simulink model "boat_dynamics_model"  (R2025a)
settings: Solver=ode4  StartTime=0.0  StopTime=15  FixedStep=Ts_sim  RelTol=1e-3
values from neighbouring files (symbols this model uses):
  ctrl_params =     [boat_controller_parameters.mat]    (also in setup_MDL.m = boat_controller_parameters())
  plant_params = boat_model_parameters_4dof()    [setup_MDL.m]
  trim =     [last_trim.mat]    (also in setup_RL.m = data.trim; tmp_trim_4dof.mat)
  u0 = u0(:)    [find_A_B_LQR.m]    (also in setup_MDL.m = trim.u0; setup_RL.m = trim.u0; tmp_continuous_controller.mat = [4.86274582601 4.86274582601 5.08309482386 4.40845063905]; tmp_discrete_augumented_LQI_controller.mat = [4.86274582601 4.86274582601 5.08309482386])
  x0 = x0(:)    [find_A_B_LQR.m]    (also in setup_MDL.m = trim.x0; setup_RL.m = trim.x0; tmp_continuous_controller.mat = [0 2.5 -0.1 0 0 0 0 0 0 0 4.86274582601 4.86274582601 ... (1; tmp_discrete_controller.mat = [0 2.5 -0.1 0 0 0 0 0 0 0 4.86274582601 4.86274582601 ... (1)
undefined symbols (not defined in the file or in its folder): Ts_sim
libraries: simulink_extras x4, sim3dlib x2, rllib x1
(part 1 of 2)
settings Model: Creator=brzan  LastModifiedBy=brzan

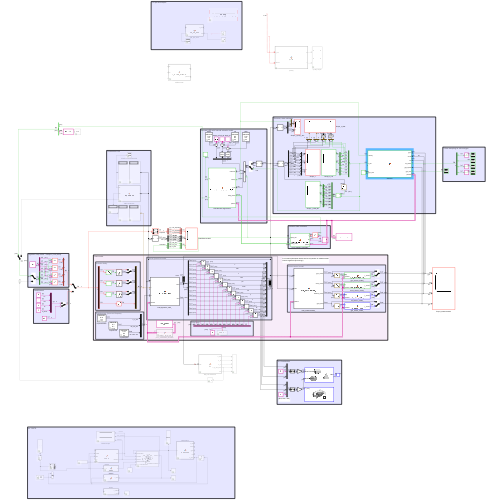
[thumbnail: Simulink's stored preview of the top-level diagram]
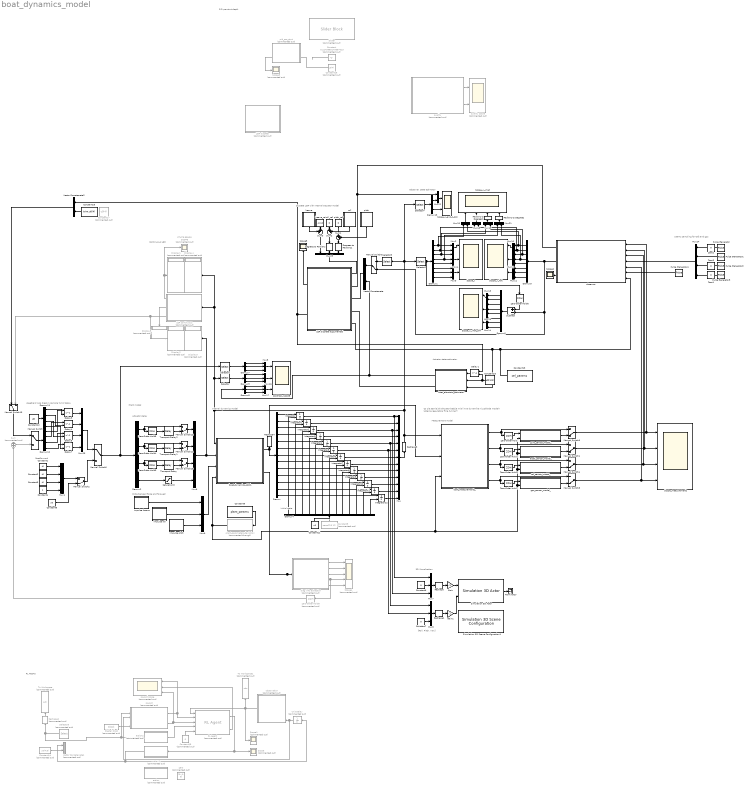
== system boat_dynamics_model ==
  note: 100ms sampling for tofs and gps
  note: Actuator state estimator
  note: PID per strut depth
  note: Plant model
  note: Actuator delay
  note: Algebraic loop break 1 sample (1ms) delay
  note: RL TESTS
  note: Observer, state estimator
  note: Co sie stanie jak aktuator bedzie mial inna dynamike niz zaklada model?
      | Uczenie regulatora (fine tuning?)
  note: Discrete LQR with Internal actuator model
  note: Continuous LQR
  note: Feedforward
  note: Measurement model
  note: Internal dynamics model
  note: Initial state
  note: Disturbances (force and forques)
  note: 3D Visualization
  note: [Roll, Pitch, Yaw]
  CONTROL SCOPE : Scope  NumInputPorts=3
      settings: ActiveDisplayYMinimum=-5.0548217064817056  ActiveDisplayYMaximum=7.8217886254018625  DataLoggingVariableName=ScopeAction
  Constant : Constant  Commented=on  Value=0.2275960170697013
  Constant1 : Constant  Value=-6
  Constant10 : Constant  Value=u0(1:3)  VectorParams1D=off
  Constant11 : Constant  Value=x0  VectorParams1D=off
  Constant12 : Constant  Value=u0  VectorParams1D=off
  Constant13 : Constant  Value=ctrl_params  VectorParams1D=off  OutDataTypeStr=Bus: ctrl_params_bus
  Constant14 : Constant  Commented=on  Value=u0(4:5)  VectorParams1D=off
  Constant15 : Constant  Commented=on  Value=0
  Constant16 : Constant  Commented=on  Value=u0(4)
  Constant17 : Constant  Commented=on  Value=u0(4)  VectorParams1D=off
  Constant18 : Constant  Value=trim.u0(4)  VectorParams1D=off
  Constant2 : Constant  Value=-6
  Constant3 : Constant  Value=-6
  Constant4 : Constant
  Constant5 : Constant  Commented=on  Value=zeros([13 1])  VectorParams1D=off
  Constant6 : Constant  Value=0
  Constant7 : Constant  Value=0
  Constant8 : Constant  Value=u0
  Constant9 : Constant  Value=plant_params  VectorParams1D=off  OutDataTypeStr=Bus: plant_params_bus
  Degrees to Radians : simulink_extras/Transformations/Degrees to Radians
  Degrees to Radians1 : simulink_extras/Transformations/Degrees to Radians
  Delay{1,3..5,7} (5 alike) : Delay  DelayLength=1  InitialConditionSource=Input port  SampleTime=Ts_sim
      settings: InputPortMap=u0,p4
  Demux : Demux  Outputs=13
  Demux1 : Demux  Outputs=8
  Demux11 : Demux
  Demux12 : Demux
  Demux13 : Demux  Outputs=2
  Demux2 : Demux
  Demux3 : Demux  Outputs=3
  Demux4 : Demux  Outputs=13
  Demux5 : Demux  Outputs=8
  Demux6 : Demux  Outputs=8
  Demux7 : Demux  Outputs=3
  Demux8 : Demux  Outputs=3
  Digital Clock : DigitalClock  Commented=on  SampleTime=0.01
  Display{1..5} (5 alike) : Display  Commented=on
  Gain : Gain  Gain=-1
  Gain1 : Gain  Gain=-1
  Impulse heave : Subsystem  mask{start=10, duration=2, amplitude=0}
      mask prompts: start "Start time"; duration "Duration time"; amplitude "Impulse amplitude"
      mask Display:
      | disp([ ...
      |     "IMPULSE"; ...
      |     'S ', ...
      |     num2str(get_param(gcb, 'start')); ...
      |     'D ', ...
      |     num2str(get_param(gcb, "duration")); ...
      |     'A ', ...
      |     num2str(get_param(gcb, "amplitude")) ...
      | ]);
  Impulse pitch : Subsystem  mask{start=10, duration=2, amplitude=0}
      mask prompts: start "Start time"; duration "Duration time"; amplitude "Impulse amplitude"
      mask Display:
      | disp([ ...
      |     "IMPULSE"; ...
      |     'S ', ...
      |     num2str(get_param(gcb, 'start')); ...
      |     'D ', ...
      |     num2str(get_param(gcb, "duration")); ...
      |     'A ', ...
      |     num2str(get_param(gcb, "amplitude")) ...
      | ]);
  Impulse roll : Subsystem  mask{start=3, duration=7, amplitude=0.5}
      mask prompts: start "Start time"; duration "Duration time"; amplitude "Impulse amplitude"
      mask Display:
      | disp([ ...
      |     "IMPULSE"; ...
      |     'S ', ...
      |     num2str(get_param(gcb, 'start')); ...
      |     'D ', ...
      |     num2str(get_param(gcb, "duration")); ...
      |     'A ', ...
      |     num2str(get_param(gcb, "amplitude")) ...
      | ]);
  Integrator : Integrator  InitialConditionSource=external  InitialCondition=-0.11
  Integrator{1,3..12} (11 alike) : Integrator  InitialConditionSource=external
  Integrator2 : Integrator  InitialConditionSource=external  InitialCondition=deg2rad(3)
  LQR continuous : MATLAB Function  Commented=on  TreatAsAtomicUnit=on
  LQR discrete : MATLAB Function  Commented=on  TreatAsAtomicUnit=on  SystemSampleTime=ctrl_params.Ts
  LQR discrete augumented : MATLAB Function  TreatAsAtomicUnit=on  SystemSampleTime=ctrl_params.Ts
  Manual Switch : ManualSwitch
  Manual Switch{1..5,8,10..12} (9 alike) : ManualSwitch  CurrentSetting=0
  Manual Switch13 : ManualSwitch
  Manual Switch6 : ManualSwitch
  Mux : Mux  Inputs=13
  Mux{1,6,23..24} (4 alike) : Mux
  Mux{2,10,13,18..22} (8 alike) : Mux  Inputs=2
  Mux{3..5,7..9,11..12,14..17,25} (13 alike) : Mux  Inputs=3
  Pulse Generator{,1..4} (5 alike) : DiscretePulseGenerator  Period=10  SampleTime=ctrl_params.Ts
  RL Agent : rllib/RL Agent  Commented=on  Agent=agentObj  ExternalActionAsInput=on  ProvideLastAction=off  ProvideCumRwd=on  TreatAsDirectFeedthrough=on  UseStrictObservationDataTypes=off
  Radians to Degrees : simulink_extras/Transformations/Radians to Degrees
  Radians to Degrees1 : simulink_extras/Transformations/Radians to Degrees
  Reshape : Reshape  OutputDimensionality=Row vector (2-D)
  Reshape1 : Reshape  OutputDimensionality=Row vector (2-D)
  Reshape2 : Reshape  Commented=on
  Reshape3 : Reshape  OutputDimensionality=Column vector (2-D)
  Reshape4 : Reshape  OutputDimensionality=Column vector (2-D)
  STATE ERROR SCOPE : Scope  Commented=on
      settings: ActiveDisplayYMinimum=-0.17004569092279864  ActiveDisplayYMaximum=0.25579071640803624  DataLoggingVariableName=ScopeData3
  Saturation3 : Saturate  UpperLimit=20  LowerLimit=0
  Scope : Scope  Commented=on
      settings: ActiveDisplayYMinimum=-2.4199088465030929  ActiveDisplayYMaximum=1.3794615097714347  DataLoggingVariableName=ScopeData2
  Scope1 : Scope  Commented=on
      settings: ActiveDisplayYMinimum=0.99404961030066707  ActiveDisplayYMaximum=1.0007752200523612  DataLoggingVariableName=ScopeData4
  Scope2 : Scope
      settings: ActiveDisplayYMinimum=-7.4600755666939691E-5  ActiveDisplayYMaximum=0.00062285522635525655  DataLoggingVariableName=ScopeData11
  Scope3 : Scope  Commented=on
      settings: ActiveDisplayYMinimum=-0.14108639149516483  ActiveDisplayYMaximum=0.0051605981146346652  DataLoggingVariableName=ScopeData12
  Scope4 : Scope  Commented=on  NumInputPorts=5
      settings: ActiveDisplayYMinimum=-0.58327189745525043  ActiveDisplayYMaximum=0.17485807514493268  DataLoggingVariableName=ScopeData13
  Scope5 : Scope
      settings: ActiveDisplayYMinimum=-0.22138752196784806  ActiveDisplayYMaximum=0.42850292012780228  DataLoggingVariableName=ScopeData6
  Scope_measurements : Scope  NumInputPorts=4
      settings: ActiveDisplayString=4  ActiveDisplayYMinimum=0.421125  ActiveDisplayYMaximum=2.9298750000000005
  Scope_x : Scope  NumInputPorts=3
      settings: ActiveDisplayYMinimum=-0.13106117710441487  ActiveDisplayYMaximum=0.06992887382000551
  Scope_x_and_z_dot : Scope  NumInputPorts=2
      settings: ActiveDisplayYMinimum=0.30889257492581745  ActiveDisplayYMaximum=2.8807711117217907  DataLoggingVariableName=ScopeData10
  Scope_x_hat : Scope  NumInputPorts=3
      settings: ActiveDisplayYMinimum=-0.12339067146341488  ActiveDisplayYMaximum=0.04600825658737881  DataLoggingVariableName=ScopeObservation
  Scope_x_xhat : Scope  NumInputPorts=4
      settings: ActiveDisplayYMinimum=-0.10922860786142216  ActiveDisplayYMaximum=-0.0926378252846192  DataLoggingVariableName=ScopeData7
  Scope_x_xhat_diff : Scope  NumInputPorts=3
      settings: ActiveDisplayYMinimum=-0.017709281074984293  ActiveDisplayYMaximum=0.023978409304645298  DataLoggingVariableName=ScopeData5
  Selector : Selector  InputPortWidth=13  IndexOptions=Index vector (dialog)  Indices=[11 12 13]  OutputSizes=1
  Selector1 : Selector  InputPortWidth=4  IndexOptions=Index vector (dialog)  Indices=[1 2 3]  OutputSizes=1
  Selector2 : Selector  InputPortWidth=13  IndexOptions=Index vector (dialog)  Indices=[3 4 5 6 7 8 9 10]  OutputSizes=1
  Selector3 : Selector  InputPortWidth=13  IndexOptions=Index vector (dialog)  Indices=[3 4 5 6 7 8 9 10]  OutputSizes=1
  Selector5 : Selector  Commented=on  InputPortWidth=5  IndexOptions=Index vector (dialog)  Indices=[1 2 3]  OutputSizes=1
  Selector7 : Selector  InputPortWidth=13  IndexOptions=Index vector (dialog)  Indices="[ 2  4 ]"  OutputSizes=1
  Simulation 3D Actor : sim3dlib/Simulation 3D Actor  Priority=1  ActorName=Boat  ParentName=Scene Origin  Operation=Create at setup  InitScriptText=|  SampleTime=-1  Translation=[0 0 0]  Rotation=[0 0 0]  Scale=[1 1 1]/1000  InputsText=Boat.Translation Boat.Rotation  aMode=5  ActorTag=Boat  ActorType=Sim3dActor  ID=C
      | % Reserved keywords:
      | % - Actor : handle to this actor object
      | % - World : handle to the world object
      | 
      | % Examples:
      | 
      | % Create a primitive geometry (optional)
      | % createShape(Actor, 'box', [1 1 1]);
      | 
      | % Initialize values (optional)
      | % Actor.Physics = true;
      | % Actor.Color = [1 0 0];
  Simulation 3D Scene Configuration1 : sim3dlib/Simulation 3D Scene Configuration  Priority=0  ProjectFormat=Default Scenes  SceneDesc=Open surface  ProjectName=C:\Program Files\MATLAB\R2025a\toolbox\shared\sim3d_projects\automotive_project_windows\UE\WindowsNoEditor\VehicleSimulation.exe  ScenePath=/Game/Maps/HwStrght  EnableOpenDRIVE=off  vehTagList={'Boat';'Custom';'Scene Origin'}  vehTag=Boat  AttachedCameraRelativeTranslation=[-4 -3 1]*1000*0.25  FreeCameraDefaultInitialTranslation=[-6, 0, 2]  AttachedCameraRelativeRotation=[0 -10 40]  FreeCameraDefaultInitialRotation=[0, -15, 0]  ViewpointName=Custom  FreeCameraInitialTranslation=[-5 0 1]  ViewpointTranslation=[0 0 0]  FreeCameraInitialRotation=[0 0 0]  ViewpointRotation=[0 0 0]  OpVisEn=off  Ts=.05  EnableWindow=on  EnableRemoteAccess=off  EnableWeather=off  SunAzimuth=90  SunAltitude=40.0  EnableGeospatialSun=off  Latitude=0  Longitude=0  Date=2023-01-01  Time=10:30:00  GeoTimeZone=-5.0  SunDaylightSaving=off  wind=1  clouds=10  EnableVolumetricClouds=off  CloudCoverage=0  CloudAltitude=6  fog=0  rain=0  RaindropsEffect=off  SnowDensity=0  EnableGeospatial=off  TilesetSource=Earth terrain  UseTrueOrigin=off  OriginHeight=200  OriginLatitude=40.744652  OriginLongitude=-73.988864  MapStyle=Aerial  AdditionalAssetIDs=[]  UseAdvancedSunSky=off  SolarTime=11  TimeZone=-5  Day=21  Month=9  Year=2022  UseDaylightSavingTime=on  DSTStartDay=10  DSTStartMonth=3  DSTEndDay=3  DSTEndMonth=11  DSTSwitchHour=2  sensorTag=MainCamera1  sensorId=1  sensorName=MainCamera1  mountLoc=Origin  offsetFlag=off  tmountOffset=[0, 0, 0]  rmountOffset=[0, 0, 0]  HorizontalResolution=1280  VerticalResolution=720  HorizontalFOV=60  mountPoint=[0 0 0]  mountOrientation=[0 0 0]  aMode=5  ID=1  GeoTrigger=Inactive  ViewNameList={'Custom'}  ViewTranslationList={'[-5 0 1]'}  ViewRotationList={'[0 0 0]'}
      settings: LibrarySourceBlock=sl3dlib/Simulation 3D/Environment/Simulation 3D Scene Configuration
  Slider : SliderBlock  Commented=on  ScaleMax=2
  Subtract : Sum  Inputs=+-
  Sum : Sum  Commented=on  Inputs=+|+
  Sum1 : Sum  Inputs=|++
  Sum2 : Sum  Inputs=|++
  Sum3 : Sum  Inputs=++|
  Terminator : Terminator
  To Workspace : ToWorkspace  Commented=on  VariableName=act  SaveFormat=Structure With Time  SampleTime=-1
  To Workspace1 : ToWorkspace  Commented=on  VariableName=obs  SaveFormat=Structure With Time  SampleTime=-1
  Transport Delay : TransportDelay  DelayTime=plant_params.hydrofoils.dynamics.L  InitialOutput=u0(3)
  Transport Delay1 : TransportDelay  DelayTime=plant_params.hydrofoils.dynamics.L  InitialOutput=u0(2)
  Transport Delay2 : TransportDelay  DelayTime=plant_params.hydrofoils.dynamics.L  InitialOutput=u0(1)
  Unit Delay : UnitDelay  Commented=on  InitialCondition=u0(1:3)  SampleTime=0.01  HasFrameUpgradeWarning=on
  Vector Concatenate : Concatenate
  Vector Concatenate1 : Concatenate  Commented=on
  Vector Concatenate2 : Concatenate
  Zero : Constant  Commented=on  Value=[0; 0; 0]  OutDataTypeStr=Inherit: Inherit via back propagation
  Zero-Order Hold : ZeroOrderHold  SampleTime=plant_params.gyro.sample_time
  Zero-Order Hold1 : ZeroOrderHold  SampleTime=plant_params.accel.sample_time
  Zero-Order Hold2 : ZeroOrderHold  SampleTime=plant_params.tof.sample_time
  Zero-Order Hold3 : ZeroOrderHold  SampleTime=plant_params.hydrofoils.dynamics.Ts_act
  Zero-Order Hold4 : ZeroOrderHold  SampleTime=plant_params.hydrofoils.dynamics.Ts_act
  Zero-Order Hold5 : ZeroOrderHold  SampleTime=plant_params.hydrofoils.dynamics.Ts_act
  Zero-Order Hold6 : ZeroOrderHold  SampleTime=ctrl_params.Ts
  Zero-Order Hold7 : ZeroOrderHold  SampleTime=plant_params.gps.sample_time
  Zero-Order Hold8 : ZeroOrderHold  Commented=on  SampleTime=0.01
  Zero1 : Constant  Value=0  OutDataTypeStr=Inherit: Inherit via back propagation
  Zero2 : Constant  Value=0  OutDataTypeStr=Inherit: Inherit via back propagation
  Zero3 : Constant  Value=0  OutDataTypeStr=Inherit: Inherit via back propagation
  accel_sensor_model_ : MATLAB Function  TreatAsAtomicUnit=on  SystemSampleTime=plant_params.accel.sample_time
  action : MATLAB Function  Commented=on  TreatAsAtomicUnit=on
  action1 : MATLAB Function  Commented=on  TreatAsAtomicUnit=on
  action2 : MATLAB Function  Commented=on  TreatAsAtomicUnit=on
  boat_actuators_estimator : MATLAB Function  TreatAsAtomicUnit=on  SystemSampleTime=ctrl_params.Ts
  boat_dynamics_4dof_ : MATLAB Function  TreatAsAtomicUnit=on
  boat_measurements_ : MATLAB Function  TreatAsAtomicUnit=on
  diag info extraction : MATLAB Function  Commented=on  TreatAsAtomicUnit=on
  gps_sensor_model_ : MATLAB Function  TreatAsAtomicUnit=on  SystemSampleTime=plant_params.tof.sample_time
  gyro_sensor_model_ : MATLAB Function  TreatAsAtomicUnit=on  SystemSampleTime=plant_params.gyro.sample_time
  heave : Subsystem  mask{start=10, duration=2, amplitude=0}
      mask prompts: start "Start time"; duration "Duration time"; amplitude "Impulse amplitude"
      mask Display:
      | disp([ ...
      |     "IMPULSE"; ...
      |     'S ', ...
      |     num2str(get_param(gcb, 'start')); ...
      |     'D ', ...
      |     num2str(get_param(gcb, "duration")); ...
      |     'A ', ...
      |     num2str(get_param(gcb, "amplitude")) ...
      | ]);
  heave_ref : Constant  Value=-0.10
  observation : MATLAB Function  Commented=on  TreatAsAtomicUnit=on  SystemSampleTime=0.01
  observer : MATLAB Function  TreatAsAtomicUnit=on  SystemSampleTime=ctrl_params.Ts
  pid_per_strut : MATLAB Function  Commented=on  TreatAsAtomicUnit=on  SystemSampleTime=ctrl_params.Ts
  pitch : Subsystem  mask{start=10, duration=2, amplitude=0}
      mask prompts: start "Start time"; duration "Duration time"; amplitude "Impulse amplitude"
      mask Display:
      | disp([ ...
      |     "IMPULSE"; ...
      |     'S ', ...
      |     num2str(get_param(gcb, 'start')); ...
      |     'D ', ...
      |     num2str(get_param(gcb, "duration")); ...
      |     'A ', ...
      |     num2str(get_param(gcb, "amplitude")) ...
      | ]);
  pitch_ref : Constant  Value=0
  plant_parameters_deviation : MATLAB Function  Commented=through  TreatAsAtomicUnit=on
  quality : MATLAB Function  Commented=on  TreatAsAtomicUnit=on  SystemSampleTime=ctrl_params.Ts
  quality scope : Scope  Commented=on  NumInputPorts=2
      settings: ActiveDisplayYMinimum=-0.12455482970730834  ActiveDisplayYMaximum=1.1240659773755071  DataLoggingVariableName=ScopeData8
  reward : MATLAB Function  Commented=on  TreatAsAtomicUnit=on  SystemSampleTime=ctrl_params.Ts
  reward scope : Scope  Commented=on  NumInputPorts=3
      settings: ActiveDisplayYMinimum=-2399.5814447480943  ActiveDisplayYMaximum=277.10834326270424  DataLoggingVariableName=ScopeData9
  roll : Subsystem  mask{start=5, duration=5, amplitude=0}
      mask prompts: start "Start time"; duration "Duration time"; amplitude "Impulse amplitude"
      mask Display:
      | disp([ ...
      |     "IMPULSE"; ...
      |     'S ', ...
      |     num2str(get_param(gcb, 'start')); ...
      |     'D ', ...
      |     num2str(get_param(gcb, "duration")); ...
      |     'A ', ...
      |     num2str(get_param(gcb, "amplitude")) ...
      | ]);
  roll_ref : Constant  Value=0
  tof_sensor_model_ : MATLAB Function  TreatAsAtomicUnit=on  SystemSampleTime=plant_params.tof.sample_time
  wires:
  boat_dynamics_4dof_/1(xdot) -> Demux/1, Reshape4/1
  Constant9/1 -> plant_parameters_deviation/1(in)
  Demux/1 -> Integrator/1
  Demux/2 -> Integrator1/1
  Demux/4 -> Integrator3/1
  Demux/3 -> Integrator2/1
  Demux/5 -> Integrator4/1
  Demux/6 -> Integrator5/1
  Integrator/1 -> Mux7/1, Mux/1  "x"
  Integrator1/1 -> Mux/2  "xdot"
  Integrator2/1 -> Mux7/3, Mux/3  "z"
  Integrator3/1 -> Mux/4  "zdot"
  Integrator4/1 -> Mux8/1, Mux/5  "phi"
  Integrator5/1 -> Mux/6, Mux8/2  "theta"
  Constant1/1 -> Mux1/1  "FL"
  Constant4/1 -> Mux1/4  "F_thrust"
  Demux1/1 -> Mux20/1, Mux2/1  "z"
  Mux2/1 -> Scope_x/1
  Demux1/2 -> Mux2/2, Mux18/1  "zdot"
  Constant3/1 -> Mux1/3  "R"
  Constant2/1 -> Mux1/2  "FR"
  Constant6/1 -> Mux7/2
  Mux8/1 -> Reshape1/1
  Mux7/1 -> Reshape/1
  Reshape/1 -> Gain/1
  Simulation 3D Actor/1 -> Terminator/1
  Gain1/1 -> Simulation 3D Actor/2
  Reshape1/1 -> Gain1/1
  Constant7/1 -> Mux8/3
  Demux/7 -> Integrator6/1
  Demux/8 -> Integrator7/1
  Integrator6/1 -> Mux/7  "ksi"
  Integrator7/1 -> Mux/8  "p"
  Demux1/3 -> Mux19/1, Mux4/1  "phi"
  Demux1/4 -> Mux21/1, Mux4/2  "theta"
  Demux1/5 -> Mux4/3  "ksi"
  Demux1/6 -> Mux3/1  "p"
  Demux1/7 -> Mux3/2  "q"
  Demux1/8 -> Mux3/3  "r"
  Mux4/1 -> Scope_x/2
  Mux3/1 -> Scope_x/3
  Manual Switch1/1 -> observer/2(accel), Scope_measurements/2  "acc"
  Manual Switch4/1 -> observer/3(tof), Scope_measurements/3  "dist"
  Zero-Order Hold/1 -> gyro_sensor_model_/1(y)
  boat_measurements_/1(gyro_vector) -> Zero-Order Hold/1, Manual Switch5/1
  Manual Switch5/1 -> observer/1(gyro), Scope_measurements/1  "gyro"
  gyro_sensor_model_/1(y_model) -> Manual Switch5/2
  boat_measurements_/3(distance_vector) -> Manual Switch4/1, Zero-Order Hold2/1
  boat_measurements_/2(accel_vector) -> Zero-Order Hold1/1, Manual Switch1/1
  Zero-Order Hold2/1 -> tof_sensor_model_/1(y)
  Zero-Order Hold1/1 -> accel_sensor_model_/1(y)
  accel_sensor_model_/1(y_model) -> Manual Switch1/2
  LQR continuous/3(u) -> Manual Switch13/2, Display2/1
  LQR continuous/2(du) -> Display5/1
  LQR continuous/1(dx) -> STATE ERROR SCOPE/1, Display1/1
  plant_parameters_deviation/1(out) -> boat_dynamics_4dof_/4(params), boat_measurements_/3(params), tof_sensor_model_/2(params), gyro_sensor_model_/2(params), accel_sensor_model_/2(params), gps_sensor_model_/2(params)
  Saturation3/1 -> Mux6/4
  Manual Switch6/1 -> Selector1/1, Demux2/1
  Demux2/3 -> Zero-Order Hold3/1, Manual Switch10/1
  Transport Delay/1 -> Manual Switch10/2
  Demux2/2 -> Manual Switch11/1, Zero-Order Hold4/1
  Transport Delay1/1 -> Manual Switch11/2
  Demux2/1 -> Manual Switch12/1, Zero-Order Hold5/1
  Transport Delay2/1 -> Manual Switch12/2
  Manual Switch10/1 -> Mux6/3
  Manual Switch11/1 -> Mux6/2
  Manual Switch12/1 -> Mux6/1
  Gain/1 -> Simulation 3D Actor/1
  Mux9/1 -> boat_dynamics_4dof_/3(w)
  Impulse heave/1(Out1) -> Mux9/1  "F_z_dist"
  Impulse roll/1(Out1) -> Mux9/2  "tau_roll_dist"
  Impulse pitch/1(Out1) -> Mux9/3  "tau_pitch_dist"
  Demux4/1 -> Integrator/2
  Demux4/8 -> Integrator7/2
  Demux4/2 -> Integrator1/2
  Demux4/3 -> Integrator2/2
  Demux4/4 -> Integrator3/2
  Demux4/5 -> Integrator4/2
  Demux4/6 -> Integrator5/2
  Demux4/7 -> Integrator6/2
  Constant11/1 -> Demux4/1
  Mux10/1 -> Scope_x_hat/1
  Mux12/1 -> Scope_x_hat/2
  Mux11/1 -> Scope_x_hat/3
  Demux5/8 -> Mux11/3  "r"
  Demux5/7 -> Mux11/2  "q"
  Demux5/6 -> Mux11/1  "p"
  Demux5/5 -> Mux12/3  "ksi"
  Demux5/4 -> Mux21/2, Mux12/2  "theta"
  Demux5/3 -> Mux19/2, Mux12/1  "phi"
  Demux5/2 -> Mux18/2, Mux10/2  "zdot"
  Demux5/1 -> Mux20/2, Mux10/1  "z"
  Mux24/1 -> observer/4(tof_status)
  Demux6/8 -> Mux14/3  "r"
  Demux6/2 -> Mux13/2  "zdot"
  Demux6/3 -> Mux15/1  "phi"
  Mux13/1 -> Scope_x_xhat_diff/1
  Demux6/1 -> Mux13/1  "z"
  Mux15/1 -> Scope_x_xhat_diff/2
  Mux14/1 -> Scope_x_xhat_diff/3
  Demux6/5 -> Mux15/3  "ksi"
  Subtract/1 -> Demux6/1
  Demux6/4 -> Mux15/2  "theta"
  Demux6/7 -> Mux14/2  "q"
  Demux6/6 -> Mux14/1  "p"
  Mux/1 -> Reshape3/1
  Manual Switch13/1 -> Manual Switch/1
  Mux23/1 -> Manual Switch6/1
  Demux/9 -> Integrator8/1
  Integrator8/1 -> Mux/9  "q"
  Integrator9/1 -> Mux/10  "r"
  Demux/10 -> Integrator9/1
  Integrator10/1 -> Mux/11  "FL"
  Demux/11 -> Integrator10/1
  Demux4/9 -> Integrator8/2
  Demux4/10 -> Integrator9/2
  Demux4/11 -> Integrator10/2
  tof_sensor_model_/1(y_model) -> Manual Switch4/2
  Demux7/2 -> Mux5/2  "FL_requested"
  Demux7/3 -> Mux5/3  "R_requested"
  Mux5/1 -> CONTROL SCOPE/1
  Demux7/1 -> Mux5/1  "FR_requested"
  Selector1/1 -> Demux7/1  "requested"
  Demux3/1 -> Mux16/1  "FR_real"
  Selector/1 -> Demux3/1  "real"
  Mux16/1 -> CONTROL SCOPE/2
  Demux3/3 -> Mux16/3  "R_real"
  Demux3/2 -> Mux16/2  "FL_real"
  Mux6/1 -> Display3/1, boat_dynamics_4dof_/2(u)
  Constant8/1 -> Manual Switch2/2
  Mux1/1 -> Manual Switch2/1
  Selector2/1 -> Zero-Order Hold6/1, Demux1/1
  Zero-Order Hold4/1 -> Transport Delay1/1
  Zero-Order Hold5/1 -> Transport Delay2/1
  Zero-Order Hold3/1 -> Transport Delay/1
  Selector3/1 -> Manual Switch3/1
  Vector Concatenate/1 -> LQR discrete augumented/3(x_hat)
  Demux8/1 -> Mux17/1  "FR_hat"
  Demux8/2 -> Mux17/2  "FL_hat"
  Mux17/1 -> CONTROL SCOPE/3
  Demux8/3 -> Mux17/3  "R_hat"
  Manual Switch3/1 -> Vector Concatenate/1
  Zero-Order Hold6/1 -> Subtract/1
  Mux19/1 -> Radians to Degrees1/1
  Mux18/1 -> Scope_x_xhat/2
  Mux20/1 -> Scope_x_xhat/1
  Mux21/1 -> Radians to Degrees/1
  Demux11/1 -> Delay3/2
  Demux12/3 -> Delay5/1
  Delay3/1 -> Mux23/1
  Demux11/2 -> Delay4/2
  Demux12/2 -> Delay4/1
  Demux12/1 -> Delay3/1
  Delay4/1 -> Mux23/2
  Demux11/3 -> Delay5/2
  Constant12/1 -> Demux11/1
  Constant13/1 -> LQR discrete augumented/5(params), boat_actuators_estimator/3(params), observer/7(params)
  reward/2(isDone) -> reward scope/3, RL Agent/3  "isDone"
  reward/1(ret) -> RL Agent/2, reward scope/1  "reward"
  observer/2(x_hat) -> Subtract/2, Manual Switch3/2, Demux5/1  "x_hat"
  Manual Switch2/1 -> Manual Switch6/2
  Constant14/1 -> Vector Concatenate1/2
  Manual Switch/1 -> Demux12/1
  Radians to Degrees/1 -> Scope_x_xhat/4
  Radians to Degrees1/1 -> Scope_x_xhat/3
  Selector5/1 -> reward/2(uLQR), action2/1(u_RL), Reshape2/1
  RL Agent/2 -> reward scope/2  "cum_reward"
  Constant15/1 -> RL Agent/5
  Delay5/1 -> Mux23/3
  Demux11/4 -> Delay7/2
  Demux12/4 -> Delay7/1
  Delay7/1 -> Mux23/4
  Reshape2/1 -> To Workspace/1
  Unit Delay/1 -> reward/3(uRL), observation/5(u_prev)
  observation/1(o) -> Scope1/1, To Workspace1/1, RL Agent/1
  RL Agent/1 -> Scope/1, action1/1(u_RL)
  Digital Clock/1 -> reward/5(time)
  action2/1(u) -> RL Agent/4
  action1/1(u) -> Unit Delay/1, Vector Concatenate1/1
  Integrator12/1 -> Mux/13  "R"
  Integrator11/1 -> Mux/12  "FR"
  Demux/12 -> Integrator11/1
  Demux4/12 -> Integrator11/2
  Demux4/13 -> Integrator12/2
  Demux/13 -> Integrator12/1
  Reshape3/1 -> Selector/1, LQR continuous/1(x), Display4/1, boat_dynamics_4dof_/1(x), Selector3/1, Selector2/1, Selector7/1, boat_measurements_/1(x)
  Selector7/1 -> Demux13/1
  Demux13/1 -> Mux22/2  "xdot"
  Demux13/2 -> Scope_x_and_z_dot/2  "zdot"
  Constant5/1 -> ?
  observer/3(gyro_bias) -> Scope2/1
  Pulse Generator/1 -> Mux24/1
  Pulse Generator1/1 -> Mux24/2
  Pulse Generator2/1 -> Mux24/3
  Pulse Generator3/1 -> Mux24/4
  Vector Concatenate2/1 -> Manual Switch13/1
  Constant/1 -> ?
  Constant16/1 -> pid_per_strut/2(vel)
  pid_per_strut/2(e) -> Scope3/1
  boat_dynamics_4dof_/2(info) -> diag info extraction/1(info)
  diag info extraction/1(F_Ds) -> Scope4/1
  diag info extraction/5(vel) -> Scope4/5
  diag info extraction/2(F_D) -> Scope4/2
  diag info extraction/3(F_T) -> Scope4/3
  Zero-Order Hold7/1 -> gps_sensor_model_/1(y)
  boat_measurements_/4(gps_speed) -> Zero-Order Hold7/1, Manual Switch8/1
  gps_sensor_model_/1(y_model) -> Manual Switch8/2
  Manual Switch8/1 -> observer/5(gps_speed), Scope_measurements/4  "gps"
  Reshape4/1 -> boat_measurements_/2(xdot)
  quality/1(Q) -> quality scope/1
  ? -> quality/1(x_hat)  "x_hat"
  quality/2(J) -> quality scope/2
  ? -> quality/2(params)
  Constant10/1 -> boat_actuators_estimator/2(u0), Delay1/2
  boat_actuators_estimator/1(alpha_hat) -> Demux8/1, Vector Concatenate/2  "estimated"
  Delay1/1 -> boat_actuators_estimator/1(u)
  LQR discrete augumented/2(u) -> Delay1/1, Vector Concatenate2/1
  Constant18/1 -> Vector Concatenate2/2
  observer/1(velocity) -> LQR discrete augumented/2(velocity), Mux22/1  "velocity"
  boat_actuators_estimator/2(delay_states) -> LQR discrete augumented/4(delay_states)
  Pulse Generator4/1 -> observer/6(gps_new)
  Mux22/1 -> Scope_x_and_z_dot/1
  diag info extraction/4(F_D_Ds_sum) -> Zero-Order Hold8/1, Scope4/4
  Demux2/4 -> Saturation3/1
  Zero-Order Hold8/1 -> Sum/2
  Sum/1 -> Manual Switch/2
  roll_ref/1 -> Sum2/1
  pitch_ref/1 -> Sum1/1
  heave_ref/1 -> Sum3/2
  Mux25/1 -> LQR discrete augumented/1(reference)
  Degrees to Radians/1 -> Mux25/2
  Degrees to Radians1/1 -> Mux25/3
  LQR discrete augumented/1(xi_) -> Scope5/1
  Sum1/1 -> Degrees to Radians1/1
  Sum2/1 -> Degrees to Radians/1
  pitch/1(Out1) -> Sum1/2
  roll/1(Out1) -> Sum2/2  "F_z_dist"
  Sum3/1 -> Mux25/1
  heave/1(Out1) -> Sum3/1

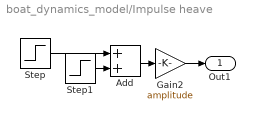
== system boat_dynamics_model/Impulse heave ==
  Add : Sum
  Gain2 : Gain  Gain=amplitude
  Step : Step  Time=start  SampleTime=0
  Step1 : Step  Time=start+duration  After=-1  SampleTime=0
  Out1 : Outport
  wires:
  Step/1 -> Add/1
  Step1/1 -> Add/2
  Gain2/1 -> Out1/1
  Add/1 -> Gain2/1

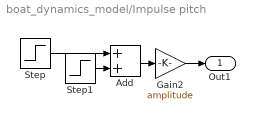
== system boat_dynamics_model/Impulse pitch ==
  Add : Sum
  Gain2 : Gain  Gain=amplitude
  Step : Step  Time=start  SampleTime=0
  Step1 : Step  Time=start+duration  After=-1  SampleTime=0
  Out1 : Outport
  wires:
  Step/1 -> Add/1
  Step1/1 -> Add/2
  Gain2/1 -> Out1/1
  Add/1 -> Gain2/1

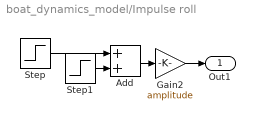
== system boat_dynamics_model/Impulse roll ==
  Add : Sum
  Gain2 : Gain  Gain=amplitude
  Step : Step  Time=start  SampleTime=0
  Step1 : Step  Time=start+duration  After=-1  SampleTime=0
  Out1 : Outport
  wires:
  Step/1 -> Add/1
  Step1/1 -> Add/2
  Gain2/1 -> Out1/1
  Add/1 -> Gain2/1

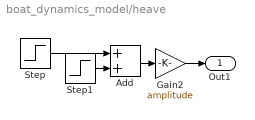
== system boat_dynamics_model/heave ==
  Add : Sum
  Gain2 : Gain  Gain=amplitude
  Step : Step  Time=start  SampleTime=0
  Step1 : Step  Time=start+duration  After=-1  SampleTime=0
  Out1 : Outport
  wires:
  Step/1 -> Add/1
  Step1/1 -> Add/2
  Gain2/1 -> Out1/1
  Add/1 -> Gain2/1

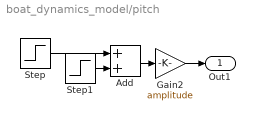
== system boat_dynamics_model/pitch ==
  Add : Sum
  Gain2 : Gain  Gain=amplitude
  Step : Step  Time=start  SampleTime=0
  Step1 : Step  Time=start+duration  After=-1  SampleTime=0
  Out1 : Outport
  wires:
  Step/1 -> Add/1
  Step1/1 -> Add/2
  Gain2/1 -> Out1/1
  Add/1 -> Gain2/1

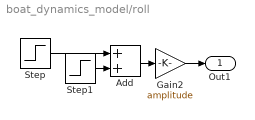
== system boat_dynamics_model/roll ==
  Add : Sum
  Gain2 : Gain  Gain=amplitude
  Step : Step  Time=start  SampleTime=0
  Step1 : Step  Time=start+duration  After=-1  SampleTime=0
  Out1 : Outport
  wires:
  Step/1 -> Add/1
  Step1/1 -> Add/2
  Gain2/1 -> Out1/1
  Add/1 -> Gain2/1

== matlab function boat_dynamics_model/plant_parameters_deviation ==
  data: in input Bus: plant_params_bus; out output Bus: plant_params_bus
function out = params_deviation(in) %#codegen
    out = in;

    % Introduce some variance
    % out.m = in.m * .8;
    % 
    % out.Ix_B = in.Ix_B * 1.2;
    % out.Iy_B = in.Iy_B * .8;
    % 
    % out.hydrofoils.dynamics.T = in.hydrofoils.dynamics.T * 1.2;
end

== matlab function boat_dynamics_model/observer ==
  data: velocity output; gyro input; x_hat output size=8; accel input; tof input; tof_status input; gps_speed input; gps_new input; params input Bus: ctrl_params_bus; gyro_bias output
function [velocity, x_hat, gyro_bias] = observer(gyro, accel, tof, tof_status, gps_speed, gps_new, params) %#codegen

    [x_hat, info] = boat_observer(gyro, accel, tof, tof_status, params);

    velocity = boat_velocity_estimator( ...
        accel, ...
        x_hat(3), ... % phi
        x_hat(4), ... % theta
        gps_speed, gps_new, ...
        params);

    gyro_bias = info.gyro_bias;
end

== matlab function boat_dynamics_model/LQR discrete ==
  data: dx output; du output; x input; u output; params input
function [dx, du, u] = lqr_discrete_controller(x, params) %#codegen
    
    % Load once (persistent)
    persistent K u0 x0 ix iu
    if isempty(K)
        data = load('tmp_discrete_controller.mat');
        K  = data.Kd;
        u0 = data.u0;
        x0 = data.x0;
        ix = data.ix;
        iu = data.iu;
    end
    
    % State error
    dx = x - x0;
    
    % LQR control
    du = -K * dx(ix);
    
    % Full control input
    u = u0;
    u(1:3) = u0(1:3) + du;   % only flap commands
end

== matlab function boat_dynamics_model/reward ==
  data: x input; uLQR input; uRL input; info input; ret output; isDone output; time input
function [ret, isDone] = reward(x, uLQR, uRL, info, time) %#codegen
    ret = 0;
    isDone = false;
    % time

    %% Unpack the x state vector
    z       = x(1);     % [m]
    z_dot   = x(2);     % [m/s]
    phi     = x(3);     % [rad]
    theta   = x(4);     % [rad]
    ksi     = x(5);     % [rad] UNUSED
    p       = x(6);     % [rad/s]
    q       = x(7);     % [rad/s]
    r       = x(8);     % [rad/s] UNUSED
    % Actuator positions
    alpha_FL = x(9);    % [deg] 
    alpha_FR = x(10);   % [deg]
    alpha_R  = x(11);   % [deg]

    %% Unpack the u and compute the error
    eFL = uLQR(1) - uRL(1); % [deg]
    eFR = uLQR(2) - uRL(2);
    eR = uLQR(3) - uRL(3);

    %% Unpack the info state vector
    z_FL = info(1);     % [m]
    z_FR = info(2);     % [m]
    z_R  = info(3);     % [m]
    V_submerged = info(4); % [m^3]
    tau_roll  = info(5);   % [Nm]
    tau_pitch = info(6);   % [Nm]   
    tau_yaw   = info(7);   % [Nm] UNUSED
    V_W       = info(8);   % [m/s]

    %% Define the parameters such as 
    % Reference
    z_ref = -0.1; % [m]
    
    % Scaling
    z_scal = 0.04; % [m]
    phi_scal   = deg2rad(4);   % [rad]
    theta_scal = deg2rad(8);   % [rad]
    p_scal     = deg2rad(64);  % [rad/s]
    q_scal     = deg2rad(128);  % [rad/s]

    % LQR scalling
    alpha_scal = 2; % [deg]

    % etc
    % V_too_deep_threshold = 0.002; % [m^3] FIXME example value

    %% Compute helpful variables
    in_water_FL = z_FL > 0.002;  % in water if z is greater than -0.002 m threshold
    in_water_FR = z_FR > 0.002;  % -0.002 
    in_water_R  = z_R  > 0.002;

    % hull_too_deep = V_submerged > V_too_deep_threshold;

    %% Compute the reward

    % Height penalty
    % ret = ret - ((z - z_ref)/z_scal)^2;
    % Attitude penalty
    % ret = ret - (phi/phi_scal)^2 - (theta/theta_scal)^2;
    % Rate penalty (damping)
    % ret = ret - (p/p_scal)^2 - (q/q_scal)^2;

    % LQR imitation error penalty
    ret = ret - ( (eFL/alpha_scal)^2 + (eFR/alpha_scal)^2 + (eR/alpha_scal)^2 );

    % If any foil near surface of water - penalty
    if ~in_water_FL || ~in_water_FR || ~in_water_R
        % ret = ret - 10;
        % ret = ret - 1;
    end

    % % If hull deep in water - penalty
    % if hull_too_deep
    %     % ret = ret - 1000; TODO FIXME
    % end

    % Reward for being alive (typical controller run costs 6400 per 1000)
    ret = ret + 60;
    % ret = ret + 100;

    %% Episode termination
    isDone = termination(x, info);

    %% Termination penalty
    if isDone 
        ret = ret -  10000 + time * 100;

        if time < 0.8
            ret = ret - 1000;
        end
    end

end

function isDone = termination(x, info) %#codege
    
    phi   = x(3);
    theta = x(4);

    z_FL = info(1);     % [m]
    z_FR = info(2);     % [m]
    z_R  = info(3);     % [m]
    V_submerged = info(4);

    isDone = false;

    % If roll > 60 deg or pitch > 40 deg 
    if abs(phi) > deg2rad(60) || abs(theta) > deg2rad(40)
        isDone = true;
    end

    % If any foil out of water - termination
    in_water_FL = z_FL > 0.0;  % in water if z is greater than -0.0 m threshold
    in_water_FR = z_FR > 0.0; 
    in_water_R  = z_R  > 0.0;

    if ~in_water_FL || ~in_water_FR || ~in_water_R
        isDone = true;
    end
    
    % % If submerged ~ 60% of volume TODO FIXME
    % if V_submerged > 0.002
    %     % isDone = true;
    % end

end

== matlab function boat_dynamics_model/action ==
  data: u_LQR input; u output; u_RL input
function u = action(u_LQR, u_RL) %#codegen
    % Residual authority [deg]
    du_max = .5;

    % Residual in degrees
    du = clamp(u_RL, -1, 1) * du_max;

    % Additive residual control
    u = u_LQR + du;
end

function y = clamp(x, lb, ub)
    y = min(max(x, lb), ub);
end

== matlab function boat_dynamics_model/quality ==
  data: x_hat input; Q output; J output; params input
function [Q, J]  = quality(x_hat, params) %#codegen

    Ts  = params.Ts;
    tau = 1;   % 2–5 s
    alpha = Ts / tau;

    % Persistent state
    persistent J_avg
    if isempty(J_avg)
        J_avg = 0;
    end

    %% Unpack the x_hat
    z       = x_hat(1);      % [m]
    z_dot   = x_hat(2);      % [m/s]
    phi     = x_hat(3);      % [rad]
    theta   = x_hat(4);      % [rad]
    % ksi unused (5)
    p       = x_hat(6);      % [rad/s]
    q       = x_hat(7);      % [rad/s]
    % r unused (8)

    %% Reference
    z_ref       = -0.1;      % [m]
    z_dot_ref   = 0.0;       % [m/s]
    phi_ref     = 0.0;       % [rad]
    theta_ref   = 0.0;       % [rad]
    p_ref       = 0.0;       % [rad/s]
    q_ref       = 0.0;       % [rad/s]

    %% Scaling (acceptable errors)
    z_scal      = 0.08;         % [m]
    z_dot_scal  = 0.10;         % [m/s]
    phi_scal    = deg2rad(5);   % [rad]
    theta_scal  = deg2rad(5);   % [rad]
    p_scal      = deg2rad(20);  % [rad/s]
    q_scal      = deg2rad(20);  % [rad/s]

    %% Calculate the penalty 
    % J = weight * (error / scale)^2
    J_tot = ...
         1 * ((z     - z_ref)     / z_scal)     ^2 + ...
         1 * ((z_dot - z_dot_ref) / z_dot_scal) ^2 + ...
         1 * ((phi   - phi_ref)   / phi_scal)   ^2 + ...
         1 * ((theta - theta_ref) / theta_scal) ^2 + ...
         1 * ((p     - p_ref)     / p_scal)     ^2 + ...
         1 * ((q     - q_ref)     / q_scal)     ^2 + ...
         0;

    % TODO add more penalty for something like hull in water
    J_tot = J_tot + 0; 

    % 1st-order LPF on J
    J_avg = J_avg + alpha * (J_tot - J_avg);
   
    %% Calculate Quality
    J_inst = J_tot;
    J_long = J_avg;

    Q_inst = exp(-J_inst);
    Q_long = exp(-J_long);

    J = [J_inst, J_long];
    Q = [Q_inst, Q_long];

end

== matlab function boat_dynamics_model/observation ==
  data: x_hat input; o output; accel input; gyro input; tof input; u_prev input
function o = observation(x_hat, accel, gyro, tof, u_prev) %#codegen
    
    z_ref = -0.1; % [m]

    %% Unpack and scale x_hat
    % z target is 0.1 i do not expect outside [0 -0.2] range but i would
    % prefer to keep the range broader a bit, by 0.1 in both directions
    % [0.1 -0.3] just in case...
    zen = clamp((x_hat(1) - z_ref) / 0.2, -1, 1);
    zdotn  = clamp(x_hat(2)/1, -1, 1); % [m/s] normalized by 

    phi   = x_hat(3);   % rad
    theta = x_hat(4);   % rad

    p_n     = clamp(x_hat(6) / deg2rad(100), -1, 1);   % rad/s normalized by 100 dps to [-1 1]
    q_n     = clamp(x_hat(7) / deg2rad(100), -1, 1);   % rad/s normalized by 100 dps to [-1 1]
    
    
    %% Unpack and scale accel
    % range is +/-2 [G]
    an = clamp(accel - [0; 0; 1] / 1.0, -1, 1); 

    %% Unpack and scale gyro
    % range is +/-2000 [dps] 
    % scaled_gyro = gyro / 2000;

    %% Unpack and scale tof
    % range is 0...255 [mm] 
    % scaled_tof = tof / 255; to 0-1 range
    % NOT USED, IT IS REDUNDANT idk?

    %% Unpack and scale control request
    % Control signal is in range -6/+12 [deg]
    % map [-6 .. +12] deg → [-1 .. +1]
    u_prev_n = (u_prev - 3.0) / 9.0;

    %% Build meaningful observation vector for the RL agent
    o = [
        zen;
        zdotn;
    
        sin(phi);
        cos(phi);
        sin(theta);
        cos(theta);
    
        p_n;
        q_n;
    
        % an(1);
        % an(2);
        an(3); % z component only xd
    
        u_prev_n(1);
        u_prev_n(2);
        u_prev_n(3)
    ];
end

function y = clamp(x, lb, ub)
    y = min(max(x, lb), ub);
end

== matlab function boat_dynamics_model/action1 ==
  data: u output; u_RL input
function u = action(u_RL) %#codegen
    u = (u_RL * 9) + 3;
end

% function y = clamp(x, lb, ub)
%     y = min(max(x, lb), ub);
% end

== matlab function boat_dynamics_model/action2 ==
  data: u output; u_RL input
function u = action(u_RL) %#codegen
    u = (u_RL - 3) / 9;
end

% function y = clamp(x, lb, ub)
%     y = min(max(x, lb), ub);
% end

== matlab function boat_dynamics_model/pid_per_strut ==
  data: x_hat input; u output; vel input; e output
function [u, e] = pid_per_strut(x_hat, vel)
%   x_hat = [
%       z;        % heave position [m]
%       z_dot;    % heave velocity [m/s]
%       phi;      % roll  [rad]
%       theta;    % pitch [rad]
%       psi;      % yaw   [rad] (unused)
%       p;        % roll rate  [rad/s]
%       q;        % pitch rate [rad/s]
%       r         % yaw rate   [rad/s] (unused)
%   ];

%% Unpack x_hat
z     = x_hat(1);
z_dot = x_hat(2);
phi   = x_hat(3);
theta = x_hat(4);
p     = x_hat(6);
q     = x_hat(7);
r     = x_hat(8);

omega_B = [p; q; r];

%% Hydrofoil positions relative to the COM
pos_front_left_B = [
    +0.216;     % [m] ahead of COM
    -0.145;     % [m] to the right of COM (negative bcs on the left)
    +0.178      % [m] below COM
]; 
pos_rear_B = [
    -0.379;     % [m] ahead of COM (negative because it is behind)
    +0.0;       % [m] to the right of COM
    +0.215      % [m] below COM
]; 
pos_front_right_B = [
    +0.216;     % [m] ahead of COM
    +0.145;     % [m] to the right of COM
    +0.178      % [m] below COM
]; 

%% Calculate each foil Z positon in world frame
cphi = cos(phi);   sphi = sin(phi);
cth  = cos(theta); sth = sin(theta);
cpsi = 1;          spsi = 0;   % yaw irrelevant for vertical, keep consistent
R_x = [1 0 0;
       0 cphi -sphi;
       0 sphi  cphi];
R_y = [ cth 0 sth;
        0   1 0;
       -sth 0 cth];
R_z = [ cpsi -spsi 0;
        spsi  cpsi 0;
        0      0   1];
R_BW = R_z * R_y * R_x;

% FRONT LEFT
r_FL_W = R_BW * pos_front_left_B;
z_FL   = z + r_FL_W(3);

v_FL_W = cross(omega_B, r_FL_W);
z_dot_FL = z_dot + v_FL_W(3);

% FRONT RIGHT
r_FR_W = R_BW * pos_front_right_B;
z_FR   = z + r_FR_W(3);

v_FR_W = cross(omega_B, r_FR_W);
z_dot_FR = z_dot + v_FR_W(3);

% REAR
r_R_W = R_BW * pos_rear_B;
z_R   = z + r_R_W(3);

v_R_W = cross(omega_B, r_R_W);
z_dot_R = z_dot + v_R_W(3);


%% PID parameters
persistent state_FL
if isempty(state_FL)
    state_FL.Kp = .000001;
    state_FL.Ki = .001;
    state_FL.Kd = .001;

    state_FL.dt = 0.01;
    state_FL.Integral = 0;
    state_FL.Integral_Limit = 0;

    state_FL.u_max = 12.0;
    state_FL.u_min = -6.0;
end
persistent state_FR
if isempty(state_FR)
    state_FR.Kp = .000001;
    state_FR.Ki = .001;
    state_FR.Kd = .001;

    state_FR.dt = 0.01;
    state_FR.Integral = 0;
    state_FR.Integral_Limit = 0;

    state_FR.u_max = 12.0;
    state_FR.u_min = -6.0;
end
persistent state_R
if isempty(state_R)
    state_R.Kp = .00001;
    state_R.Ki = .001;
    state_R.Kd = .001;

    state_R.dt = 0.01;
    state_R.Integral = 0;
    state_R.Integral_Limit = 0;

    state_R.u_max = 12.0;
    state_R.u_min = -6.0;
end

%% Desired COM above the water is z = -100 (z=0 com at water level z<0 com above water)
% So each wing should be at pos_ - [0; 0; 100]_B 

z_ref = -.100;

e_z_FL = (pos_front_left_B(3) + z_ref) - z_FL;
e_z_dot_FL = -z_dot_FL;

e_z_FR = (pos_front_right_B(3) + z_ref) - z_FR;
e_z_dot_FR = -z_dot_FR;

e_z_R  = (pos_rear_B(3) + z_ref) - z_R;
e_z_dot_R  = -z_dot_R;

%% Call each controller on each position error
[alpha_FL, state_FL] = pid(state_FL, e_z_FL, e_z_dot_FL);
[alpha_FR, state_FR] = pid(state_FR, e_z_FR, e_z_dot_FR);
[alpha_R,  state_R]  = pid(state_R,  e_z_R,  e_z_dot_R);


%% Output calculated angles
% u = [
%     alpha_FL;   % front left
%     alpha_FR;   % front right
%     alpha_R;   % rear
%     vel
% ];

u = [
    alpha_FL;   % front left
    alpha_FR;   % front right
    7;   % rear
    vel
];


% Output error
e = [e_z_FL; e_z_FR; e_z_R];

end

function [u, state] = pid(state, e, e_dot)

    % Integration
    state.Integral = state.Integral + e * state.dt;
    
    % Anti windup
    if state.Integral_Limit ~= 0
        state.Integral = min( ...
            max(state.Integral, -state.Integral_Limit), ...
            state.Integral_Limit);
    end
    
    % P I D calculation and summation
    u = state.Kp * e + ...
        state.Ki * state.Integral + ...
        state.Kd * e_dot;

    % Output saturation
    u = min(max(u, state.u_min), state.u_max);
end

== matlab function boat_dynamics_model/diag info extraction ==
  data: info input; F_Ds output; F_D output; F_T output; F_D_Ds_sum output; vel output
function [F_Ds, F_D, F_T, F_D_Ds_sum, vel] = fcn(info)

% F_Ds_FL = info.F_Ds_R;
% F_Ds_FR = info.F_Ds_FR;
% F_Ds_R = info.F_Ds_R;

F_Ds_FL = info(9);
F_Ds_FR = info(10);
F_Ds_R  = info(11);

F_D_FL = info(12);
F_D_FR = info(13);
F_D_R  = info(14);

%%
F_Ds = [F_Ds_FL, F_Ds_FR, F_Ds_R];
F_D = [F_D_FL, F_D_FR, F_D_R];
F_T = info(15);

F_D_Ds_sum = (F_Ds_FL + F_Ds_FR + F_Ds_R + F_D_FL + F_D_FR + F_D_R);

vel = info(8);

== matlab function boat_dynamics_model/gps_sensor_model_ ==
  data: y input; y_model output; params input
function y_model = gps_sensor_model_(y, params) %#codegen

    % Unpack the parameters
    noise_sigma = params.gps.noise_sigma;
    quantization_step = params.gps.quantization_step;
    
    % Assert dimensions
    assert(isscalar(y));
    assert(isscalar(noise_sigma));
    assert(isscalar(quantization_step) && (quantization_step > 0));

    % Add white noise
    y_model = y + noise_sigma .* randn(size(y));

    % Ground speed cannot be negative
    y_model = abs(y_model);

    % Quantize
    y_model = quantization_step .* round(y_model ./ quantization_step);
end

== matlab function boat_dynamics_model/boat_dynamics_4dof_ ==
  data: x input; xdot output size=[13,1]; u input; w input; params input size=1; info output
function [ xdot, info ] = boat_dynamics_4dof_(x, u, w, params) %#codegen

    [ xdot, info ] = boat_dynamics_4dof(x, u, w, params);

end

== matlab function boat_dynamics_model/boat_measurements_ ==
  data: x input; xdot input; gyro_vector output; params input; accel_vector output; distance_vector output; gps_speed output
function [ gyro_vector, accel_vector, distance_vector, gps_speed ] = boat_measurements_(x, xdot, params) %#codegen
    [ gyro_vector, accel_vector, distance_vector, gps_speed ] = boat_measurements(x, xdot, params);
end

== matlab function boat_dynamics_model/gyro_sensor_model_ ==
  data: y input; y_model output; params input
function y_model = gyro_sensor_model_(y, params) %#codegen

    % Unpack the parameters
    noise_sigma = params.gyro.noise_sigma;
    bias = params.gyro.bias;
    % bias = [0.048; 0.082; -0.173];
    % bias = [0; 0; 0];
    range_dps = params.gyro.range_dps;
    quantization_step = params.gyro.quantization_step;
    
    % Assert dimensions
    assert(isequal(size(y), [3 1]));
    assert(isequal(size(noise_sigma), [3 1]));
    assert(isequal(size(bias), [3 1]));
    assert(isscalar(range_dps) && (range_dps > 0));
    assert(isscalar(quantization_step) && (quantization_step > 0));

    % Add white noise
    y_model = y + noise_sigma .* randn(size(y));

    % Add bias
    y_model = y_model + bias;

    % Saturate to allowed sensor range
    y_model = min(max(y_model, -range_dps), range_dps);

    % Quantize
    y_model = quantization_step .* round(y_model ./ quantization_step);
end

== matlab function boat_dynamics_model/boat_actuators_estimator ==
  data: u input size=3; alpha_hat output size=3; u0 input; params input; delay_states output size=[12 1]
function [alpha_hat, delay_states] = boat_actuators_estimator(u, u0, params) %#codegen
    
    [alpha_hat, delay_states] = boat_actuators_estimator(u, u0, params);

end

== matlab function boat_dynamics_model/accel_sensor_model_ ==
  data: y input; y_model output; params input
function y_model = accel_sensor_model_(y, params) %#codegen

    % Unpack the parameters
    noise_sigma = params.accel.noise_sigma;
    range_g = params.accel.range_g;
    quantization_step = params.accel.quantization_step;
    
    % Assert dimensions
    assert(isequal(size(y), [3 1]));
    assert(isequal(size(noise_sigma), [3 1]));
    assert(isscalar(range_g) && (range_g > 0));
    assert(isscalar(quantization_step) && (quantization_step > 0));

    % Add white noise
    y_model = y + noise_sigma .* randn(size(y));

    % Saturate to allowed sensor range
    y_model = min(max(y_model, -range_g), range_g);

    % Quantize
    y_model = quantization_step .* round(y_model ./ quantization_step);
end

== matlab function boat_dynamics_model/tof_sensor_model_ ==
  data: y input; y_model output; params input
function y_model = tof_sensor_model_(y, params) %#codegen

    % Unpack the parameters
    noise_sigma_a = params.tof.noise_sigma_a;
    noise_sigma_b = params.tof.noise_sigma_b;
    range_mm_min = params.tof.range_mm_min;
    range_mm_max = params.tof.range_mm_max;
    quantization_step = params.tof.quantization_step;
    
    % Assert dimensions
    assert(isequal(size(y), [4 1]));
    assert(isscalar(noise_sigma_a));
    assert(isscalar(noise_sigma_b));
    assert(isscalar(range_mm_min));
    assert(isscalar(range_mm_max));
    assert(range_mm_min < range_mm_max);
    assert(isscalar(quantization_step) && (quantization_step > 0));

    % Noise is linearly dependant on distance
    noise_sigma = noise_sigma_a .* y + noise_sigma_b;

    % Add white noise
    y_model = y + noise_sigma .* randn(size(y));

    % Saturate to allowed sensor range
    y_model = min(max(y_model, range_mm_min), range_mm_max);

    % Quantize
    y_model = quantization_step .* round(y_model ./ quantization_step);
end
